simulink model "PPM"  (R2020a)
settings: Solver=VariableStepAuto  StartTime=0.0  StopTime=0.11  RelTol=1e-3
libraries: powerlib_meascontrol x2, simulink x1
settings Model: Creator=Naeem Mohammad  LastModifiedBy=Naeem Mohammad

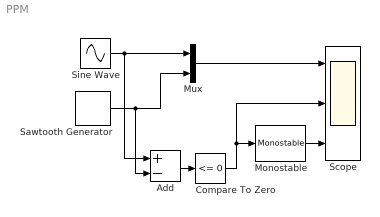
== system PPM ==
  Add : Sum  Inputs=+-
  Compare To Zero : simulink/Logic and Bit Operations/Compare To Zero  relop=<=  OutDataTypeStr=boolean
  Monostable : powerlib_meascontrol/Logic/Monostable  EdgeDetect=Rising  PulseDuration=0.002  ic=0  Ts=0
      settings: SourceProductBaseCode=PS
  Mux : Mux  Inputs=2
  Sawtooth Generator : powerlib_meascontrol/Pulse & Signal Generators/Sawtooth Generator  Freq=60  Phase=180  Ts=0
  Scope : Scope  NumInputPorts=3
  Sine Wave : Sin  Amplitude=0.75  Frequency=60  SampleTime=0
  wires:
  Add/1 -> Compare To Zero/1
  Sine Wave/1 -> Mux/1, Add/1
  Sawtooth Generator/1 -> Mux/2, Add/2
  Mux/1 -> Scope/1
  Compare To Zero/1 -> Monostable/1, Scope/2
  Monostable/1 -> Scope/3
